simulink library "tqd"  (R2021b)
settings: Solver=VariableStepAuto  StartTime=0.0  StopTime=10.0  RelTol=1e-3
undefined symbols (not defined in the file or in its folder): ATQD_AccelLimitInRange_X_rpm, ATQD_AccelLimitInRange_Y_Nm, ATQD_AccelLimitOvrKi_X_Nm, ATQD_AccelLimitOvrKp_X_Nm, ATQD_BOSMapD_X_rpm, ATQD_BOSMapD_Y_pct, ATQD_BOSMapR_X_rpm, ATQD_BOSMapR_Y_pct, ATQD_HVBCurrSmooth_X_A, ATQD_LHMTqMapDLC_X_rpm, ATQD_LHMTqMapDLC_Y_pct, ATQD_LHMTqMapRLC_X_rpm, ATQD_LHMTqMapRLC_Y_pct, ATQD_NormalMapDLC_X_rpm, ATQD_NormalMapDLC_Y_pct, ATQD_NormalTqDecSR_X_rpm, ATQD_NormalTqDecSR_Y_Nm, ATQD_NormalTqIncSR_X_rpm, ATQD_NormalTqIncSR_Y_Nm, ATQD_OPDMapRLC_X_rpm, ATQD_OPDMapRLC_Y_pct, ATQD_RollRegTorReq_X_rpm, ATQD_RollRegTorReq_Y_enum, ATQD_VehSpdLimitInRange_X_rpm, ATQD_VehSpdLimitInRange_Y_Nm, ATQD_VehSpdLimitOvrKi_X_Nm, ATQD_VehSpdLimitOvrKp_X_Nm, EIGHT_INT, ENUM_BRAKEPEDAL_PRESSED, ENUM_BRAKEPEDAL_RELEASED, ENUM_COMBOKEY_DOWN, ENUM_COMBOKEY_M1, ENUM_COMBOKEY_M2, ENUM_COMBOKEY_NONE, ENUM_COMBOKEY_RKNEE, ENUM_COMBOKEY_STOPLV, ENUM_COMBOKEY_UP, ENUM_CP2VKNEEREQ_REQUEST, ENUM_CP2VNLVREQ_LEVEL1, ENUM_CP2VNLVREQ_LEVEL2, ENUM_CP2VNLVREQ_LOWER, ENUM_CP2VNLVREQ_STOPLV, ENUM_CP2VNLVREQ_UPPER, ENUM_CREEPIND_DISABLE, ENUM_CREEPIND_READY, ENUM_CREEPIND_RUNNING, ENUM_CREEPIND_WARNING, ENUM_DRIVELINERELEASE_RELEASE, ENUM_EBSTORQUERWQ_LIMIT, ENUM_EBSTORQUERWQ_TORQUE, ENUM_ECPVCUDRM_CONFORT, ENUM_ECPVCUDRM_ECO, ENUM_ECPVCUDRM_NORMAL, ENUM_ECPVCUDRM_NOTAVAILABLE, ENUM_EMTqModeDrvBrk_Accel, ENUM_EMTqModeDrvBrk_Brake, ENUM_EMTqModeDrvBrk_Coast, ENUM_ETC2ACTDRIVEDIR_BACKWARD, ENUM_ETC2ACTDRIVEDIR_FORWARD, ENUM_ETC2ACTDRIVEDIR_STILL ... (+341)
libraries: simulink x109, hcu_lib x67
(part 1 of 13)
settings Model: Creator=13615  LastModifiedBy=zack
settings SolverCC: AlgebraicLoopSolver=TrustRegion
settings DataIOCC: SaveFormat=Array  SignalLoggingSaveFormat=ModelDataLogs  ReturnWorkspaceOutputs=off
settings OptimizationCC: BlockReduction=off  BooleanDataType=off
settings DebuggingCC: SaveWithParameterizedLinksMsg=none  UnderspecifiedInitializationDetection=Classic  MergeDetectMultiDrivingBlocksExec=none  SignalResolutionControl=TryResolveAllWithWarning
settings HardwareCC: TargetUnknown=on
settings ModelReferenceCC: PropagateSignalLabelsOutOfModel=off
settings SFSimCC: SimUseLocalCustomCode=off
settings RTWCC: RTWUseLocalCustomCode=off
settings ConfigComp: CovMetricSettings=dw  CovSaveCumulativeToWorkspaceVar=on  CovSaveSingleToWorkspaceVar=on

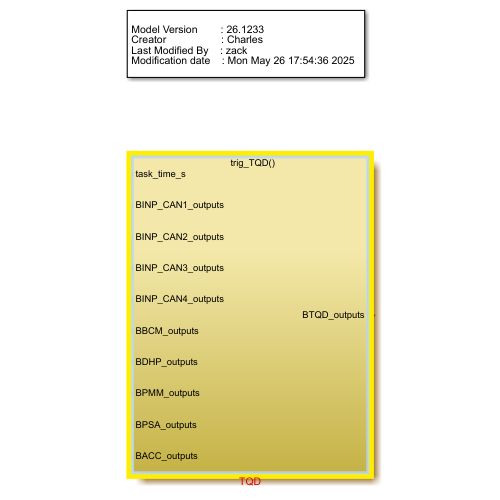
[thumbnail: Simulink's stored preview of the top-level diagram]
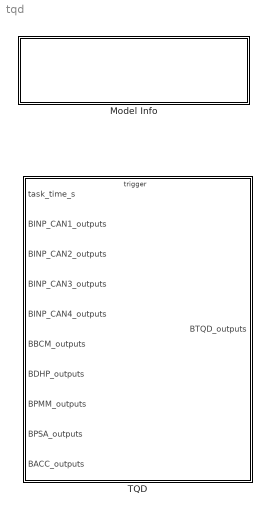
== system tqd ==
  Model Info : Subsystem  LoadFcn=slcm LoadBlock;  InitFcn=slcm('UpdateAllCMBlocksInThisModelInit')  mask(CMBlock){InitialSaveTempField=, InitialBlockCM=None, BlockCM=None, Frame=on, SaveTempField=, DisplayStringWithTags=|, MaskDisplayString=Model Version        : 26.1236\nCreator                   : Charles\nLast Modified By    : zack\nModification date    : Mon May 26 18:16:00 2025, HorizontalTextAlignment=Left, LeftAlignmentValue=0.02, SourceBlockDiagram=tqd, TagMaxNumber=20, CMTag1=, CMTag2=, CMTag3=, CMTag4=, CMTag5=, CMTag6=, CMTag7=, CMTag8=, CMTag9=, CMTag10=, CMTag11=, CMTag12=, CMTag13=, CMTag14=, CMTag15=, CMTag16=, CMTag17=, CMTag18=, CMTag19=, CMTag20=}
      mask DisplayStringWithTags=|
      | Model Version        : %<ModelVersion>
      | Creator                   : Charles
      | Last Modified By    : %<LastModifiedBy>
      | Modification date    : %<LastModificationDate>
      mask help: This block allows revision control information to be displayed within the model.
      settings: CopyFcn=slcm CopyBlock;  DeleteFcn=slcm Cancel;  PostSaveFcn=slcm('UpdateAllCMBlocksInThisModel')  NameChangeFcn=slcm Rename;  OpenFcn=slcm
      mask Display: text(str2num(LeftAlignmentValue), 0.5, MaskDisplayString, 'HorizontalAlignment', HorizontalTextAlignment)
  TQD : Subsystem
      settings: RTWSystemCode=Nonreusable function  RTWFcnNameOpts=Use subsystem name  RTWFileNameOpts=Use subsystem name

== system tqd/Model Info ==
  EmptySubsystem : Subsystem

== system tqd/TQD ==
  task_time_s : Inport  OutDataTypeStr=single
  BINP_CAN1_outputs : Inport  Port=2  OutDataTypeStr=Bus:BINP_CAN1_outputs
  BINP_CAN2_outputs : Inport  Port=3  OutDataTypeStr=Bus: BINP_CAN2_outputs
  BINP_CAN3_outputs : Inport  Port=4  OutDataTypeStr=Bus:BINP_CAN3_outputs
  BINP_CAN4_outputs : Inport  Port=5  OutDataTypeStr=Bus:BINP_CAN4_outputs
  BBCM_outputs : Inport  Port=6  OutDataTypeStr=Bus:BBCM_outputs
  BDHP_outputs : Inport  Port=7  OutDataTypeStr=Bus:BDHP_outputs
  BPMM_outputs : Inport  Port=8  OutDataTypeStr=Bus:BPMM_outputs
  BPSA_outputs : Inport  Port=9  OutDataTypeStr=Bus:BPSA_outputs
  BACC_outputs : Inport  Port=10  OutDataTypeStr=Bus:BACC_outputs
  trig_TQD : TriggerPort  TriggerType=function-call  VariantControl=(inherit)
  Input_Convert : Subsystem
      settings: RTWSystemCode=Nonreusable function
  Main : Subsystem
      settings: RTWSystemCode=Nonreusable function
  OutpConvert : Subsystem
      settings: RTWSystemCode=Nonreusable function
  SCP_In : Subsystem
      settings: RTWSystemCode=Nonreusable function
  SCP_Out : Subsystem
      settings: RTWSystemCode=Nonreusable function
  BTQD_outputs : Outport  OutDataTypeStr=Bus:BTQD_outputs
  wires:
  task_time_s/1 -> SCP_In/1(task_time_s)
  BINP_CAN1_outputs/1 -> SCP_In/2(BINP_CAN1_outputs)
  BINP_CAN2_outputs/1 -> SCP_In/3(BINP_CAN2_outputs)
  BINP_CAN3_outputs/1 -> SCP_In/4(BINP_CAN3_outputs)
  BINP_CAN4_outputs/1 -> SCP_In/5(BINP_CAN4_outputs)
  BBCM_outputs/1 -> SCP_In/6(BBCM_outputs)
  BDHP_outputs/1 -> SCP_In/7(BDHP_outputs)
  BPMM_outputs/1 -> SCP_In/8(BPMM_outputs)
  BPSA_outputs/1 -> SCP_In/9(BPSA_outputs)
  SCP_In/1(BSCPIn_outputs) -> [BSCPIn_outputs]
  [BSCPIn_outputs] -> Input_Convert/1(BSCPIn_outputs)
  [BMain_outputs] -> Input_Convert/2(BMain_outputs)
  Input_Convert/1(BInpConvert_outputs) -> [BInpConvert_outputs]
  [BInpConvert_outputs] -> Main/2(BInpConvert_outputs)
  [BSCPIn_outputs] -> Main/1(BSCPIn_outputs)
  Main/1(BMain_outputs) -> [BMain_outputs]
  [BSCPIn_outputs] -> OutpConvert/1(BSCPIn_outputs)
  [BInpConvert_outputs] -> OutpConvert/2(BInpConvert_outputs)
  [BMain_outputs] -> OutpConvert/3(BMain_outputs)
  OutpConvert/1(BOutpConvert_outputs) -> [BOutpConvert_outputs]
  [BMain_outputs] -> SCP_Out/2(BMain_outputs)
  [BOutpConvert_outputs] -> SCP_Out/3(BOutpConvert_outputs)
  [BInpConvert_outputs] -> SCP_Out/1(BInpConvert_outputs)
  SCP_Out/1(BTQD_outputs) -> BTQD_outputs/1
  BACC_outputs/1 -> SCP_In/10(BACC_outputs)

== system tqd/Model Info/EmptySubsystem ==

== system tqd/TQD/Input_Convert ==
  BSCPIn_outputs : Inport
  BMain_outputs : Inport  Port=2
  Bus Creator : BusCreator  Inputs=101
  Bus Selector : BusSelector  OutputSignals=VTQD_AccelPedalDepressed_flg,VTQD_BrkSWOn_flg,VTQD_DoorOpen_flg,VTQD_DrivePositionOn_flg,VTQD_NeutralPositionOn_flg,VTQD_ReversePositionOn_flg,VTQD_EVDriveReady_flg,VTQD_IGNActive_flg,VTQD_EM1ReqTorqLimDriv_Nm,VTQD_EM1ReqTorqLimBrk_Nm,VTQD_ActFRDoorOPSta_flg,VTQD_ActMDDoorOPSta_flg,VTQD_ActTDDoorOPSta_flg,VTQD_VCU4PweLmtInd_flg,VTQD_GearFlashIndDis_flg,VTQD_GearFlashInd_flg,VTQD_EVCU1VehActDrvDir_enum,VTQD_VCUMCUDemHiPosVal_rpm,VTQD_SpdLimSta_flg,VTQD_EngModeEnDetTime_s,VTQD_EngModeEnDetEnd_flg,VTQD_LVchrgSvrMode_flg,VTQD_EngModeDisDetTime_s,VTQD_EngModeDisDetEnd_flg,VTQD_AmberFlashOn_flg,VTQD_AmberFlashOff_flg,VTQD_Function1Off_flg,VTQD_Function2Off_flg,VTQD_Function3Off_flg,VTQD_Function4Off_flg,VTQD_Function5Off_flg,VTQD_ComboKeyEn_flg,VTQD_ComboKeyPreEn_flg,VTQD_FunctionOffSta_enum,VTQD_LostComBCU_flg,VTQD_LostComDMS_flg,VTQD_LostComEBS_flg,VTQD_LostComTempEBS_flg,VTQD_LostComTempMCU_flg,VTQD_LostComTempBCU_flg,VTQD_SpdForceZero_flg,VTQD_TrqForceZero_flg,VTQD_TrqLimit_flg,VTQD_SpdLimit_flg,VTQD_DMSLossLimitGear_flg,VTQD_DRTransfer_flg,VTQD_TMRotateDirectionReq_enum,VTQD_ActvDmpDisabReq_flg,VTQD_ForceDischarge_flg,VTQD_TqTargetShaftSpd_rpm,VTQD_PTAvailMotTq_Nm,VTQD_PTAvailGenTq_Nm,VTQD_ActDriveMode_enum,VTQD_ComLostZeroPwr_flg,VTQD_EBSLostZeroReg_flg,VTQD_ActCAN1BUSOFF_flg,VTQD_EM1LimitCtrlBrk_flg,VTQD_EM1TorqueCtrlBrk_flg,VTQD_EM1TorqueCtrlDriv_flg,VTQD_EM1LimitCtrlDriv_flg,VTQD_TrqCMDForveZero_flg,VTQD_TqSource_enum,VTQD_TMSpd_rpm,VTQD_VCUTMVehSpd_kph,VTQD_VCUVehSpd_kph
  Bus Selector1 : BusSelector  OutputSignals=VTQD_GearActualPosn_enum,VTQD_ParkingPawlPwrOn_flg,VTQD_ParkingPawlEnable_flg,VTQD_TorqLimDoorOpn_flg,VTQD_VCUMCUCtrlMdTQD_enum,VTQD_PedalMapTq_Nm,VTQD_BOSTqDecRate_pct,VTQD_CreepSpdReq_rpm,VTQD_CreepStart_flg,VTQD_CreepIND_enum,VTQD_ActTUpAIND_enum,VTQD_VCUEBSHHSw_enum,VTQD_VCUEBSRd4BR_enum,VTQD_TUpADisableCreep_flg,VTQD_RollingRegenEnable_flg,VTQD_RollRegTorReq_Nm,VTQD_VehSpdLimitEnable_flg,VTQD_VehSpdLimitTG_kph,VTQD_VehSpdTorLimit_Nm,VTQD_VehAcclLimitEnable_flg,VTQD_VehAcclLimitTG_mps2,VTQD_VehAcclTorLimit_Nm,VTQD_VehAccel_mps2,VTQD_ParkingProtectWarning_flg,VTQD_ParkingProtectAction_flg,VTQD_TqCMDUpLim_Nm,VTQD_TqCMDLowLim_Nm,VTQD_RampTs_c,VTQD_RampTqIncSR_Nm,VTQD_RampTqDecSR_Nm,VTQD_FrEDUSpRat_rat,VTQD_RrEDUSpRat_rat,VTQD_FinalTrqUpLim_Nm,VTQD_FinalTrqLowLim_Nm,VTQD_TMTqCapMot_Nm,VTQD_TMTqCapGen_Nm
  Function : Subsystem
      settings: RTWSystemCode=Nonreusable function
  Input Signal Convert : Subsystem
      settings: RTWSystemCode=Nonreusable function
  BInpConvert_outputs : Outport
  wires:
  BSCPIn_outputs/1 -> [BSCPIn_outputs]
  BMain_outputs/1 -> [BMain_outputs]
  [BSCPIn_outputs] -> Input Signal Convert/1(BSCPIn_outputs)
  Input Signal Convert/1(BSignalConvert_outputs) -> [BSignalConvert_outputs]
  [BSCPIn_outputs] -> Function/1(BSCPIn_outputs)
  [BSignalConvert_outputs] -> Function/2(BSignalConvert_outputs)
  [BMain_outputs] -> Input Signal Convert/3(BDCQ_main_outputs)
  [BMain_outputs] -> Function/3(BMain_outputs)
  Function/1(BFunction_outputs) -> [BFunction_outputs]
  [BFunction_outputs] -> Input Signal Convert/2(BDCQ_Function_outputs)
  [BSignalConvert_outputs] -> Bus Selector/1
  [BFunction_outputs] -> Bus Selector1/1
  Bus Selector/1 -> Bus Creator/1  "<VTQD_AccelPedalDepressed_flg>"
  Bus Selector/2 -> Bus Creator/2  "<VTQD_BrkSWOn_flg>"
  Bus Selector/3 -> Bus Creator/3  "<VTQD_DoorOpen_flg>"
  Bus Selector/4 -> Bus Creator/4  "<VTQD_DrivePositionOn_flg>"
  Bus Selector/5 -> Bus Creator/5  "<VTQD_NeutralPositionOn_flg>"
  Bus Selector/6 -> Bus Creator/6  "<VTQD_ReversePositionOn_flg>"
  Bus Selector/7 -> Bus Creator/7  "<VTQD_EVDriveReady_flg>"
  Bus Selector/8 -> Bus Creator/8  "<VTQD_IGNActive_flg>"
  Bus Selector/9 -> Bus Creator/9  "<VTQD_EM1ReqTorqLimDriv_Nm>"
  Bus Selector/10 -> Bus Creator/10  "<VTQD_EM1ReqTorqLimBrk_Nm>"
  Bus Selector/11 -> Bus Creator/11  "<VTQD_ActFRDoorOPSta_flg>"
  Bus Selector/12 -> Bus Creator/12  "<VTQD_ActMDDoorOPSta_flg>"
  Bus Selector/13 -> Bus Creator/13  "<VTQD_ActTDDoorOPSta_flg>"
  Bus Selector/14 -> Bus Creator/14  "<VTQD_VCU4PweLmtInd_flg>"
  Bus Selector/15 -> Bus Creator/15  "<VTQD_GearFlashIndDis_flg>"
  Bus Selector/16 -> Bus Creator/16  "<VTQD_GearFlashInd_flg>"
  Bus Selector/17 -> Bus Creator/17  "<VTQD_EVCU1VehActDrvDir_enum>"
  Bus Selector/18 -> Bus Creator/18  "<VTQD_VCUMCUDemHiPosVal_rpm>"
  Bus Selector/19 -> Bus Creator/19  "<VTQD_SpdLimSta_flg>"
  Bus Selector/20 -> Bus Creator/20  "<VTQD_EngModeEnDetTime_s>"
  Bus Selector/21 -> Bus Creator/21  "<VTQD_EngModeEnDetEnd_flg>"
  Bus Selector/22 -> Bus Creator/22  "<VTQD_LVchrgSvrMode_flg>"
  Bus Selector/23 -> Bus Creator/23  "<VTQD_EngModeDisDetTime_s>"
  Bus Selector/24 -> Bus Creator/24  "<VTQD_EngModeDisDetEnd_flg>"
  Bus Selector/25 -> Bus Creator/25  "<VTQD_AmberFlashOn_flg>"
  Bus Selector/26 -> Bus Creator/26  "<VTQD_AmberFlashOff_flg>"
  Bus Selector/27 -> Bus Creator/27  "<VTQD_Function1Off_flg>"
  Bus Selector/28 -> Bus Creator/28  "<VTQD_Function2Off_flg>"
  Bus Selector/29 -> Bus Creator/29  "<VTQD_Function3Off_flg>"
  Bus Selector/30 -> Bus Creator/30  "<VTQD_Function4Off_flg>"
  Bus Selector/31 -> Bus Creator/31  "<VTQD_Function5Off_flg>"
  Bus Selector/32 -> Bus Creator/32  "<VTQD_ComboKeyEn_flg>"
  Bus Selector/33 -> Bus Creator/33  "<VTQD_ComboKeyPreEn_flg>"
  Bus Selector/34 -> Bus Creator/34  "<VTQD_FunctionOffSta_enum>"
  Bus Selector/35 -> Bus Creator/35  "<VTQD_LostComBCU_flg>"
  Bus Selector/36 -> Bus Creator/36  "<VTQD_LostComDMS_flg>"
  Bus Selector/37 -> Bus Creator/37  "<VTQD_LostComEBS_flg>"
  Bus Selector/38 -> Bus Creator/38  "<VTQD_LostComTempEBS_flg>"
  Bus Selector/39 -> Bus Creator/39  "<VTQD_LostComTempMCU_flg>"
  Bus Selector/40 -> Bus Creator/40  "<VTQD_LostComTempBCU_flg>"
  Bus Selector/41 -> Bus Creator/41  "<VTQD_SpdForceZero_flg>"
  Bus Selector/42 -> Bus Creator/42  "<VTQD_TrqForceZero_flg>"
  Bus Selector/43 -> Bus Creator/43  "<VTQD_TrqLimit_flg>"
  Bus Selector/44 -> Bus Creator/44  "<VTQD_SpdLimit_flg>"
  Bus Selector/45 -> Bus Creator/45  "<VTQD_DMSLossLimitGear_flg>"
  Bus Selector/46 -> Bus Creator/46  "<VTQD_DRTransfer_flg>"
  Bus Selector/47 -> Bus Creator/47  "<VTQD_TMRotateDirectionReq_enum>"
  Bus Selector/48 -> Bus Creator/48  "<VTQD_ActvDmpDisabReq_flg>"
  Bus Selector/49 -> Bus Creator/49  "<VTQD_ForceDischarge_flg>"
  Bus Selector/50 -> Bus Creator/50  "<VTQD_TqTargetShaftSpd_rpm>"
  Bus Selector/51 -> Bus Creator/51  "<VTQD_PTAvailMotTq_Nm>"
  Bus Selector/52 -> Bus Creator/52  "<VTQD_PTAvailGenTq_Nm>"
  Bus Selector/53 -> Bus Creator/53  "<VTQD_ActDriveMode_enum>"
  Bus Selector/54 -> Bus Creator/54  "<VTQD_ComLostZeroPwr_flg>"
  Bus Selector/55 -> Bus Creator/55  "<VTQD_EBSLostZeroReg_flg>"
  Bus Selector/56 -> Bus Creator/56  "<VTQD_ActCAN1BUSOFF_flg>"
  Bus Selector/57 -> Bus Creator/57  "<VTQD_EM1LimitCtrlBrk_flg>"
  Bus Selector/58 -> Bus Creator/58  "<VTQD_EM1TorqueCtrlBrk_flg>"
  Bus Selector/59 -> Bus Creator/59  "<VTQD_EM1TorqueCtrlDriv_flg>"
  Bus Selector/60 -> Bus Creator/60  "<VTQD_EM1LimitCtrlDriv_flg>"
  Bus Selector/61 -> Bus Creator/61  "<VTQD_TrqCMDForveZero_flg>"
  Bus Selector/62 -> Bus Creator/62  "<VTQD_TqSource_enum>"
  Bus Selector/63 -> Bus Creator/63  "<VTQD_TMSpd_rpm>"
  Bus Selector/64 -> Bus Creator/64  "<VTQD_VCUTMVehSpd_kph>"
  Bus Selector/65 -> Bus Creator/65  "<VTQD_VCUVehSpd_kph>"
  Bus Selector1/9 -> Bus Creator/74  "<VTQD_CreepStart_flg>"
  Bus Selector1/8 -> Bus Creator/73  "<VTQD_CreepSpdReq_rpm>"
  Bus Selector1/10 -> Bus Creator/75  "<VTQD_CreepIND_enum>"
  Bus Selector1/7 -> Bus Creator/72  "<VTQD_BOSTqDecRate_pct>"
  Bus Selector1/11 -> Bus Creator/76  "<VTQD_ActTUpAIND_enum>"
  Bus Selector1/6 -> Bus Creator/71  "<VTQD_PedalMapTq_Nm>"
  Bus Selector1/12 -> Bus Creator/77  "<VTQD_VCUEBSHHSw_enum>"
  Bus Selector1/5 -> Bus Creator/70  "<VTQD_VCUMCUCtrlMdTQD_enum>"
  Bus Selector1/13 -> Bus Creator/78  "<VTQD_VCUEBSRd4BR_enum>"
  Bus Selector1/4 -> Bus Creator/69  "<VTQD_TorqLimDoorOpn_flg>"
  Bus Selector1/14 -> Bus Creator/79  "<VTQD_TUpADisableCreep_flg>"
  Bus Selector1/3 -> Bus Creator/68  "<VTQD_ParkingPawlEnable_flg>"
  Bus Selector1/15 -> Bus Creator/80  "<VTQD_RollingRegenEnable_flg>"
  Bus Selector1/2 -> Bus Creator/67  "<VTQD_ParkingPawlPwrOn_flg>"
  Bus Selector1/16 -> Bus Creator/81  "<VTQD_RollRegTorReq_Nm>"
  Bus Selector1/1 -> Bus Creator/66  "<VTQD_GearActualPosn_enum>"
  Bus Selector1/17 -> Bus Creator/82  "<VTQD_VehSpdLimitEnable_flg>"
  Bus Selector1/18 -> Bus Creator/83  "<VTQD_VehSpdLimitTG_kph>"
  Bus Selector1/19 -> Bus Creator/84  "<VTQD_VehSpdTorLimit_Nm>"
  Bus Selector1/20 -> Bus Creator/85  "<VTQD_VehAcclLimitEnable_flg>"
  Bus Selector1/21 -> Bus Creator/86  "<VTQD_VehAcclLimitTG_mps2>"
  Bus Selector1/22 -> Bus Creator/87  "<VTQD_VehAcclTorLimit_Nm>"
  Bus Selector1/23 -> Bus Creator/88  "<VTQD_VehAccel_mps2>"
  Bus Selector1/24 -> Bus Creator/89  "<VTQD_ParkingProtectWarning_flg>"
  Bus Selector1/25 -> Bus Creator/90  "<VTQD_ParkingProtectAction_flg>"
  Bus Selector1/26 -> Bus Creator/91  "<VTQD_TqCMDUpLim_Nm>"
  Bus Selector1/27 -> Bus Creator/92  "<VTQD_TqCMDLowLim_Nm>"
  Bus Selector1/28 -> Bus Creator/93  "<VTQD_RampTs_c>"
  Bus Selector1/29 -> Bus Creator/94  "<VTQD_RampTqIncSR_Nm>"
  Bus Selector1/30 -> Bus Creator/95  "<VTQD_RampTqDecSR_Nm>"
  Bus Selector1/31 -> Bus Creator/96  "<VTQD_FrEDUSpRat_rat>"
  Bus Selector1/32 -> Bus Creator/97  "<VTQD_RrEDUSpRat_rat>"
  Bus Selector1/33 -> Bus Creator/98  "<VTQD_FinalTrqUpLim_Nm>"
  Bus Selector1/34 -> Bus Creator/99  "<VTQD_FinalTrqLowLim_Nm>"
  Bus Selector1/35 -> Bus Creator/100  "<VTQD_TMTqCapMot_Nm>"
  Bus Selector1/36 -> Bus Creator/101  "<VTQD_TMTqCapGen_Nm>"
  Bus Creator/1 -> BInpConvert_outputs/1  "BInpConvert_outputs"

== system tqd/TQD/Main ==
  BSCPIn_outputs : Inport
  BInpConvert_outputs : Inport  Port=2
  Available Torqeu Limitation : Subsystem
      settings: RTWSystemCode=Nonreusable function
  Bus Creator : BusCreator  Inputs=9
  Driver Torque Demmand : Subsystem
      settings: RTWSystemCode=Nonreusable function
  Gear Ratio : Subsystem
  Motor Direction : Subsystem
      settings: RTWSystemCode=Nonreusable function
  Ramp Input Torque : Subsystem
      settings: RTWSystemCode=Nonreusable function
  Torque Coordination : Subsystem
      settings: RTWSystemCode=Nonreusable function
  Torque Distribution : Subsystem
      settings: RTWSystemCode=Nonreusable function
  Torque Ramp : Subsystem
      settings: RTWSystemCode=Nonreusable function
  BMain_outputs : Outport
  wires:
  [VTQD_TMTqReq_Nm] -> Bus Creator/9
  Ramp Input Torque/1(VTQD_RrRampInpTqRr_Nm) -> [VTQD_RrRampInpTqRr_Nm]
  [VTQD_RrRampInpTqRr_Nm] -> Torque Ramp/3(VTQD_RrRampInpTqRr_Nm)
  [BInpConvert_outputs] -> Torque Distribution/1(BInpConvert_outputs)
  Torque Distribution/1(VTQD_CoorTqDemFr_Nm) -> [VTQD_CoorTqDemFr_Nm]
  [BSCPIn_outputs] -> Available Torqeu Limitation/2(BSCPIn_outputs)
  Bus Creator/1 -> BMain_outputs/1  "BMain_outputs"
  [VTQD_AfterAvailableTqDemRr_Nm] -> Bus Creator/5
  [VTQD_DriverTqDem_Nm] -> Torque Coordination/2(VTQD_DriverTqDem_Nm)
  [VTQD_TMTqReqRaw_Nm] -> Motor Direction/2(VTQD_TMTqReqRaw_Nm)
  [BInpConvert_outputs] -> Ramp Input Torque/1(BInpConvert_outputs)
  Motor Direction/1(VTQD_TMTqReq_Nm) -> [VTQD_TMTqReq_Nm]
  Torque Ramp/2(VTQD_RrRampTq_Nm) -> [VTQD_RrRampTq_Nm]
  [BSCPIn_outputs] -> Ramp Input Torque/2(BSCPIn_outputs)
  Torque Distribution/2(VTQD_CoorTqDemRr_Nm) -> [VTQD_CoorTqDemRr_Nm]
  Torque Ramp/1(VTQD_TMTqReqRaw_Nm) -> [VTQD_TMTqReqRaw_Nm]
  [VTQD_CoordTqDem_Nm] -> Bus Creator/2
  [BInpConvert_outputs] -> Motor Direction/1(BInpConvert_outputs)
  [VTQD_RrRampInpTqRr_Nm] -> Bus Creator/6
  [VTQD_RrRampTq_Nm] -> Bus Creator/8
  [VTQD_DriverTqDem_Nm] -> Bus Creator/1
  [VTQD_CoorTqDemRr_Nm] -> Available Torqeu Limitation/3(VTQD_CoorTqDemRr_Nm)
  [VTQD_CoorTqDemRr_Nm] -> Bus Creator/4
  BSCPIn_outputs/1 -> [BSCPIn_outputs]
  [BInpConvert_outputs] -> Torque Coordination/1(BInpConvert_outputs)
  Torque Coordination/1(VTQD_CoordTqDem_Nm) -> [VTQD_CoordTqDem_Nm]
  [BInpConvert_outputs] -> Driver Torque Demmand/1(BDCQ_InpConvert_outputs)
  [BInpConvert_outputs] -> Available Torqeu Limitation/1(BInpConvert_outputs)
  Driver Torque Demmand/1(VTQD_DriverTqDem_Nm) -> [VTQD_DriverTqDem_Nm]
  BInpConvert_outputs/1 -> [BInpConvert_outputs]
  [VTQD_CoordTqDem_Nm] -> Torque Distribution/2(VTQD_CoordTqDem_Nm)
  [VTQD_AfterAvailableTqDemRr_Nm] -> Ramp Input Torque/3(VTQD_AfterAvailableTqDemRr_Nm)
  [BInpConvert_outputs] -> Torque Ramp/1(BInpConvert_outputs)
  Available Torqeu Limitation/1(VTQD_AfterAvailableTqDemRr_Nm) -> [VTQD_AfterAvailableTqDemRr_Nm]
  [VTQD_CoorTqDemFr_Nm] -> Bus Creator/3
  [VTQD_TMTqReqRaw_Nm] -> Bus Creator/7
  [BSCPIn_outputs] -> Torque Ramp/2(BSCPIn_outputs)

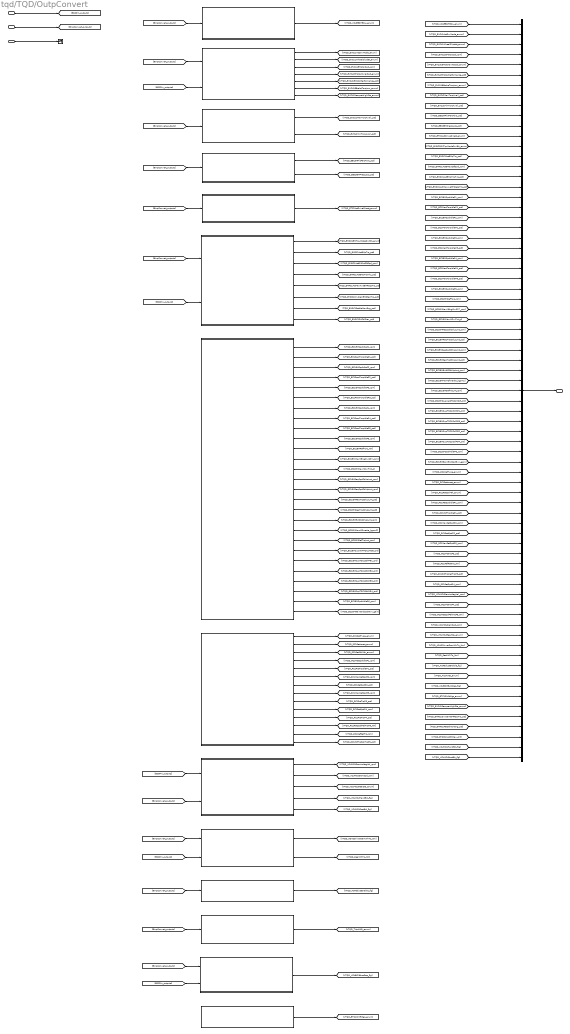
== system tqd/TQD/OutpConvert ==
  BSCPIn_outputs : Inport
  BInpConvert_outputs : Inport  Port=2
  BMain_outputs : Inport  Port=3
  ABS_System_Enable : Subsystem
      settings: RTWSystemCode=Nonreusable function
  ADAS_DriverWheelTqDem : Subsystem
      settings: RTWSystemCode=Nonreusable function
  Bus Creator : BusCreator  Inputs=73
  Buzzer Request : Subsystem
      settings: RTWSystemCode=Nonreusable function
  EC1 SCP : Subsystem
      settings: RTWSystemCode=Nonreusable function
  EEC3 SCP : Subsystem
      settings: RTWSystemCode=Nonreusable function
  EMRC1 SCP : Subsystem
      settings: RTWSystemCode=Nonreusable function
  ETC1 SCP : Subsystem
      settings: RTWSystemCode=Nonreusable function
  ETC2 SCP : Subsystem
      settings: RTWSystemCode=Nonreusable function
  EVCU1 SCP : Subsystem
      settings: RTWSystemCode=Nonreusable function
  EVCU2 SCP : Subsystem
      settings: RTWSystemCode=Nonreusable function
  MCUCMD SCP : Subsystem
      settings: RTWSystemCode=Nonreusable function
  MSF SCP : Subsystem
      settings: RTWSystemCode=Nonreusable function
  RC1 SCP : Subsystem
      settings: RTWSystemCode=Nonreusable function
  TUpA Indication : Subsystem
      settings: RTWSystemCode=Nonreusable function
  Terminator : Terminator
  BOutpConvert_outputs : Outport
  wires:
  [VTQD_EC1PercTorqIdleP4_pct] -> Bus Creator/25
  [BSCPIn_outputs] -> EVCU1 SCP/2(BSCPIn_outputs)
  [VTQD_RC1RetSpdP4_rpm] -> Bus Creator/56
  [VTQD_EC1EMGainEndSpdGvn_gain] -> Bus Creator/44
  MSF SCP/1(VTQD_VCUEBSHBSw_enum) -> [VTQD_VCUEBSHBSw_enum]
  [VTQD_EVCU2MaxTorqAvail_pct] -> Bus Creator/8
  EVCU1 SCP/4(VTQD_EVCU1EMotorOvrerSpd_enum) -> [VTQD_EVCU1EMotorOvrerSpd_enum]
  BInpConvert_outputs/1 -> [BInpConvert_outputs]
  EVCU1 SCP/2(VTQD_EVCU1WheelSlipdet_enum) -> [VTQD_EVCU1WheelSlipdet_enum]
  [VTQD_EC1EMSpdIdleP5_rpm] -> Bus Creator/27
  [BInpConvert_outputs] -> MSF SCP/1(BInpConvert_outputs)
  [BInpConvert_outputs] -> ETC2 SCP/1(BInpConvert_outputs)
  [VTQD_EC1EMSupTSC1CtrlPG2_cnt] -> Bus Creator/41
  [BInpConvert_outputs] -> EVCU1 SCP/1(BInpConvert_outputs)
  EC1 SCP/13(VTQD_EC1EMMaxMOvrTmt_s) -> [VTQD_EC1EMMaxMOvrTmt_s]
  [VTQD_RealWhTq_Nm] -> Bus Creator/63
  EVCU1 SCP/1(VTQD_EVCU1ActDrvMode_enum) -> [VTQD_EVCU1ActDrvMode_enum]
  [VTQD_EC1EMSupTSC1CtrlPG3_cnt] -> Bus Creator/40
  BSCPIn_outputs/1 -> [BSCPIn_outputs]
  [BInpConvert_outputs] -> EVCU2 SCP/1(BInpConvert_outputs)
  [VTQD_EVCU1WheelSlipdet_enum] -> Bus Creator/3
  EVCU1 SCP/3(VTQD_EVCU1EMotorSpd_rpm) -> [VTQD_EVCU1EMotorSpd_rpm]
  [BSCPIn_outputs] -> EMRC1 SCP/2(BSCPIn_outputs)
  [VTQD_VCUMCUDemLoNegVal_rpm] -> Bus Creator/57
  EC1 SCP/10(VTQD_EC1EMSpdIdleP5_rpm) -> [VTQD_EC1EMSpdIdleP5_rpm]
  [BInpConvert_outputs] -> EEC3 SCP/1(BInpConvert_outputs)
  [VTQD_EC1EMReqSpdCtrlUpLmt_rpm] -> Bus Creator/33
  [VTQD_EC1EMSpdIdleP2_rpm] -> Bus Creator/20
  EC1 SCP/25(VTQD_EC1EMSupTSC1CtrlPG4_cnt) -> [VTQD_EC1EMSupTSC1CtrlPG4_cnt]
  EMRC1 SCP/3(VTQD_EMRC1ActEMOutSftSpd_rpm) -> [VTQD_EMRC1ActEMOutSftSpd_rpm]
  RC1 SCP/14(VTQD_RC1PctTrqPekTrqP5_pct) -> [VTQD_RC1PctTrqPekTrqP5_pct]
  EC1 SCP/7(VTQD_EC1EMSpdIdleP4_rpm) -> [VTQD_EC1EMSpdIdleP4_rpm]
  EEC3 SCP/1(VTQD_EEC3NFricPercTorq_pct) -> [VTQD_EEC3NFricPercTorq_pct]
  EC1 SCP/22(VTQD_EC1EMSupTSC1CtrlPG1_cnt) -> [VTQD_EC1EMSupTSC1CtrlPG1_cnt]
  EEC3 SCP/2(VTQD_EEC3EMPressLoss_pct) -> [VTQD_EEC3EMPressLoss_pct]
  EMRC1 SCP/1(VTQD_EMRC1EMTquModeDrvBrk_enum) -> [VTQD_EMRC1EMTquModeDrvBrk_enum]
  [VTQD_EC1EMMaxMOvrTmt_s] -> Bus Creator/30
  [VTQD_EC1EMExtRSCtrlUpLmt_rpm] -> Bus Creator/35
  EC1 SCP/1(VTQD_EC1EMSpdIdleP1_rpm) -> [VTQD_EC1EMSpdIdleP1_rpm]
  [VTQD_EVCU1EMotorOvrerSpd_enum] -> Bus Creator/5
  [BInpConvert_outputs] -> EMRC1 SCP/1(BInpConvert_outputs)
  [BSCPIn_outputs] -> MCUCMD SCP/1(BSCPIn_outputs)
  EMRC1 SCP/2(VTQD_EMRC1ActEMpTrq_pct) -> [VTQD_EMRC1ActEMpTrq_pct]
  EVCU1 SCP/5(VTQD_EVCU1EMotorPerformance_pct) -> [VTQD_EVCU1EMotorPerformance_pct]
  [VTQD_RC1MaxRetSpdP3_rpm] -> Bus Creator/52
  [VTQD_RC1RetLocat_enum] -> Bus Creator/46
  [VTQD_ETC2ActDriveDirect_enum] -> Bus Creator/12
  EC1 SCP/3(VTQD_EC1EMSpdIdleP2_rpm) -> [VTQD_EC1EMSpdIdleP2_rpm]
  [VTQD_EC1PercTorqIdleP2_pct] -> Bus Creator/21
  [VTQD_RC1RetSpdP2_pct] -> Bus Creator/51
  [VTQD_EC1EMSpdIdleP3_rpm] -> Bus Creator/22
  EC1 SCP/14(VTQD_EC1EMReqSpdCtrlLoLmt_rpm) -> [VTQD_EC1EMReqSpdCtrlLoLmt_rpm]
  EVCU2 SCP/2(VTQD_EVCU2MinTorqAvail_pct) -> [VTQD_EVCU2MinTorqAvail_pct]
  RC1 SCP/13(VTQD_RC1RefRetTrq_Nm) -> [VTQD_RC1RefRetTrq_Nm]
  [VTQD_EMRC1ActEMOutSftSpd_rpm] -> Bus Creator/15
  [VTQD_EMRC1EMTquModeDrvBrk_enum] -> Bus Creator/13
  [VTQD_EC1PercTorqIdleP5_pct] -> Bus Creator/26
  [VTQD_EMRC1ActEMpTrq_pct] -> Bus Creator/14
  [VTQD_EC1EMReqSpdCtrlLoLmt_rpm] -> Bus Creator/31
  [BInpConvert_outputs] -> ABS_System_Enable/1(BInpConvert_outputs)
  ADAS_DriverWheelTqDem/1(VTQD_ADASDriverDemWhTq_Nm) -> [VTQD_ADASDriverDemWhTq_Nm]
  RC1 SCP/4(VTQD_RC1RetSpdIdleP1_rpm) -> [VTQD_RC1RetSpdIdleP1_rpm]
  EC1 SCP/8(VTQD_EC1PercTorqIdleP4_pct) -> [VTQD_EC1PercTorqIdleP4_pct]
  [VTQD_EC1EMSupTSC1CtrlPG4_cnt] -> Bus Creator/42
  [VTQD_RC1PctTrqIdleP1_pct] -> Bus Creator/49
  [VTQD_EC1EMMaxMEngOvrSP7_rpm] -> Bus Creator/29
  [VTQD_RC1PctTrqPekTrqP5_pct] -> Bus Creator/55
  BMain_outputs/1 -> Terminator/1
  [VTQD_RC1RetSpdIdleP1_rpm] -> Bus Creator/48
  RC1 SCP/8(VTQD_RC1MaxRetSpdP3_rpm) -> [VTQD_RC1MaxRetSpdP3_rpm]
  MCUCMD SCP/3(VTQD_VCUMCUGearSta_enum) -> [VTQD_VCUMCUGearSta_enum]
  [BSCPIn_outputs] -> Buzzer Request/2(BSCPIn_outputs)
  EC1 SCP/4(VTQD_EC1PercTorqIdleP2_pct) -> [VTQD_EC1PercTorqIdleP2_pct]
  EC1 SCP/27(VTQD_EC1EMGainEndSpdGvn_gain) -> [VTQD_EC1EMGainEndSpdGvn_gain]
  [VTQD_EC1EMReqTrqCtrlUpLmt_pct] -> Bus Creator/34
  [VTQD_EC1EMSpdHdleP6_rpm] -> Bus Creator/43
  EMRC1 SCP/5(VTQD_EMRC1ActMaxAvaEMRecpTrq_pct) -> [VTQD_EMRC1ActMaxAvaEMRecpTrq_pct]
  [VTQD_RC1PctTrqP4_pct] -> Bus Creator/58
  [BInpConvert_outputs] -> Buzzer Request/1(BInpConvert_outputs)
  RC1 SCP/11(VTQD_RC1PctTrqP4_pct) -> [VTQD_RC1PctTrqP4_pct]
  [VTQD_VCUMCUGearSta_enum] -> Bus Creator/61
  EC1 SCP/20(VTQD_EC1EMDefTrqLmt_rpm) -> [VTQD_EC1EMDefTrqLmt_rpm]
  [VTQD_EEC3NFricPercTorq_pct] -> Bus Creator/10
  [VTQD_RC1RetSpdPekTrqP5_Nm] -> Bus Creator/59
  [VTQD_RC1PctTrqP3_pct] -> Bus Creator/53
  [VTQD_EC1EMRefTorq_Nm] -> Bus Creator/28
  [VTQD_ADASDriverDemWhTq_Nm] -> Bus Creator/62
  [VTQD_RC1RetCtrlMth_enum] -> Bus Creator/47
  [BInpConvert_outputs] -> TUpA Indication/1(BInpConvert_outputs)
  [VTQD_VCUMCUDemSpd_rpm] -> Bus Creator/60
  [VTQD_EMRC1ActMaxAvaEMRecpTrq_pct] -> Bus Creator/17
  [VTQD_RC1MaxRetSpdP2_rpm] -> Bus Creator/50
  EVCU1 SCP/6(VTQD_EVCU1EBrakeTorqLow_enum) -> [VTQD_EVCU1EBrakeTorqLow_enum]
  [VTQD_EC1PercTorqIdleP1_pct] -> Bus Creator/19
  [VTQD_EC1PercTorqIdleP3_pct] -> Bus Creator/23
  [VTQD_EC1EMSpdIdleP4_rpm] -> Bus Creator/24
  [VTQD_RC1RefRetTrq_Nm] -> Bus Creator/54
  [VTQD_TqReductEnable_flg] -> Bus Creator/64
  [VTQD_EC1EMDefTrqLmt_rpm] -> Bus Creator/37
  [VTQD_RC1RetType_enum] -> Bus Creator/45
  [VTQD_EC1EMMomOfInertia_kgpm2] -> Bus Creator/36
  [BSCPIn_outputs] -> ADAS_DriverWheelTqDem/2(BSCPIn_outputs)
  [VTQD_TUpAIND_enum] -> Bus Creator/65
  [VTQD_EC1EMSupTSC1CtrlPG1_cnt] -> Bus Creator/39
  Bus Creator/1 -> BOutpConvert_outputs/1  "BOutpConvert_outputs"
  [VTQD_EC1EMSupVarRTSC1MSG_cnt] -> Bus Creator/38
  [VTQD_EC1EMReqTrqCtrlLoLmt_pct] -> Bus Creator/32
  [VTQD_VCUBCMBuzzReq_flg] -> Bus Creator/66
  EC1 SCP/12(VTQD_EC1EMMaxMEngOvrSP7_rpm) -> [VTQD_EC1EMMaxMEngOvrSP7_rpm]
  EMRC1 SCP/4(VTQD_EMRC1ActEMpTrqHrls_pct) -> [VTQD_EMRC1ActEMpTrqHrls_pct]
  [VTQD_EVCU1EBrakeTorqLow_enum] -> Bus Creator/7
  RC1 SCP/1(VTQD_RC1RetType_enum) -> [VTQD_RC1RetType_enum]
  [VTQD_EVCU1EMotorSpd_rpm] -> Bus Creator/4
  RC1 SCP/10(VTQD_RC1RetSpdP4_rpm) -> [VTQD_RC1RetSpdP4_rpm]
  [VTQD_EVCU1EMotorPerformance_pct] -> Bus Creator/6
  MCUCMD SCP/1(VTQD_VCUMCUDemLoNegVal_rpm) -> [VTQD_VCUMCUDemLoNegVal_rpm]
  EC1 SCP/16(VTQD_EC1EMReqTrqCtrlLoLmt_pct) -> [VTQD_EC1EMReqTrqCtrlLoLmt_pct]
  RC1 SCP/12(VTQD_RC1RetSpdPekTrqP5_Nm) -> [VTQD_RC1RetSpdPekTrqP5_Nm]
  [VTQD_EEC3EMPressLoss_pct] -> Bus Creator/11
  [VTQD_EVCU1ActDrvMode_enum] -> Bus Creator/2
  [VTQD_VCUEBSHBSw_enum] -> Bus Creator/1
  Buzzer Request/1(VTQD_VCUBCMBuzzReq_flg) -> [VTQD_VCUBCMBuzzReq_flg]
  [VTQD_EVCU2MinTorqAvail_pct] -> Bus Creator/9
  [VTQD_EC1EMSpdIdleP1_rpm] -> Bus Creator/18
  [VTQD_EMRC1ActEMpTrqHrls_pct] -> Bus Creator/16
  EC1 SCP/6(VTQD_EC1PercTorqIdleP3_pct) -> [VTQD_EC1PercTorqIdleP3_pct]
  EC1 SCP/9(VTQD_EC1PercTorqIdleP5_pct) -> [VTQD_EC1PercTorqIdleP5_pct]
  EC1 SCP/11(VTQD_EC1EMRefTorq_Nm) -> [VTQD_EC1EMRefTorq_Nm]
  EC1 SCP/15(VTQD_EC1EMReqSpdCtrlUpLmt_rpm) -> [VTQD_EC1EMReqSpdCtrlUpLmt_rpm]
  ETC2 SCP/1(VTQD_ETC2ActDriveDirect_enum) -> [VTQD_ETC2ActDriveDirect_enum]
  EC1 SCP/17(VTQD_EC1EMReqTrqCtrlUpLmt_pct) -> [VTQD_EC1EMReqTrqCtrlUpLmt_pct]
  EC1 SCP/23(VTQD_EC1EMSupTSC1CtrlPG2_cnt) -> [VTQD_EC1EMSupTSC1CtrlPG2_cnt]
  EC1 SCP/24(VTQD_EC1EMSupTSC1CtrlPG3_cnt) -> [VTQD_EC1EMSupTSC1CtrlPG3_cnt]
  EC1 SCP/26(VTQD_EC1EMSpdHdleP6_rpm) -> [VTQD_EC1EMSpdHdleP6_rpm]
  EC1 SCP/18(VTQD_EC1EMExtRSCtrlUpLmt_rpm) -> [VTQD_EC1EMExtRSCtrlUpLmt_rpm]
  RC1 SCP/3(VTQD_RC1RetCtrlMth_enum) -> [VTQD_RC1RetCtrlMth_enum]
  EC1 SCP/5(VTQD_EC1EMSpdIdleP3_rpm) -> [VTQD_EC1EMSpdIdleP3_rpm]
  EC1 SCP/21(VTQD_EC1EMSupVarRTSC1MSG_cnt) -> [VTQD_EC1EMSupVarRTSC1MSG_cnt]
  RC1 SCP/5(VTQD_RC1PctTrqIdleP1_pct) -> [VTQD_RC1PctTrqIdleP1_pct]
  EC1 SCP/2(VTQD_EC1PercTorqIdleP1_pct) -> [VTQD_EC1PercTorqIdleP1_pct]
  [BInpConvert_outputs] -> ADAS_DriverWheelTqDem/1(BInpConvert_outputs)
  RC1 SCP/7(VTQD_RC1RetSpdP2_pct) -> [VTQD_RC1RetSpdP2_pct]
  MCUCMD SCP/2(VTQD_VCUMCUDemSpd_rpm) -> [VTQD_VCUMCUDemSpd_rpm]
  EVCU2 SCP/1(VTQD_EVCU2MaxTorqAvail_pct) -> [VTQD_EVCU2MaxTorqAvail_pct]
  RC1 SCP/6(VTQD_RC1MaxRetSpdP2_rpm) -> [VTQD_RC1MaxRetSpdP2_rpm]
  RC1 SCP/9(VTQD_RC1PctTrqP3_pct) -> [VTQD_RC1PctTrqP3_pct]
  ADAS_DriverWheelTqDem/2(VTQD_RealWhTq_Nm) -> [VTQD_RealWhTq_Nm]
  RC1 SCP/2(VTQD_RC1RetLocat_enum) -> [VTQD_RC1RetLocat_enum]
  EC1 SCP/19(VTQD_EC1EMMomOfInertia_kgpm2) -> [VTQD_EC1EMMomOfInertia_kgpm2]
  ABS_System_Enable/1(VTQD_TqReductEnable_flg) -> [VTQD_TqReductEnable_flg]
  TUpA Indication/1(VTQD_TUpAIND_enum) -> [VTQD_TUpAIND_enum]
  ETC1 SCP/1(VTQD_ETC1ShiftrPgs_enum) -> [VTQD_ETC1ShiftrPgs_enum]
  [VTQD_ETC1ShiftrPgs_enum] -> Bus Creator/67
  EVCU1 SCP/7(VTQD_EVCU1RecuperHighSta_enum) -> [VTQD_EVCU1RecuperHighSta_enum]
  [VTQD_EVCU1RecuperHighSta_enum] -> Bus Creator/68
  EMRC1 SCP/6(VTQD_EMRC1DrvDemEMRtapTrq_pct) -> [VTQD_EMRC1DrvDemEMRtapTrq_pct]
  EMRC1 SCP/7(VTQD_EMRC1RetSelNonEng_pct) -> [TQD_EMRC1RetSelNonEng_pct]
  EMRC1 SCP/8(VTQD_EMRC1SACtrlDev_cnt) -> [VTQD_EMRC1SACtrlDev_cnt]
  [VTQD_EMRC1DrvDemEMRtapTrq_pct] -> Bus Creator/69
  [TQD_EMRC1RetSelNonEng_pct] -> Bus Creator/70
  [VTQD_EMRC1SACtrlDev_cnt] -> Bus Creator/71
  [BInpConvert_outputs] -> MCUCMD SCP/2(BInpConvert_outputs)
  MCUCMD SCP/4(VTQD_VCUMCUHandBrk_flg) -> [VTQD_VCUMCUHandBrk_flg]
  MCUCMD SCP/5(VTQD_VCUMCUFootBrk_flg) -> [VTQD_VCUMCUFootBrk_flg]
  [VTQD_VCUMCUHandBrk_flg] -> Bus Creator/72
  [VTQD_VCUMCUFootBrk_flg] -> Bus Creator/73

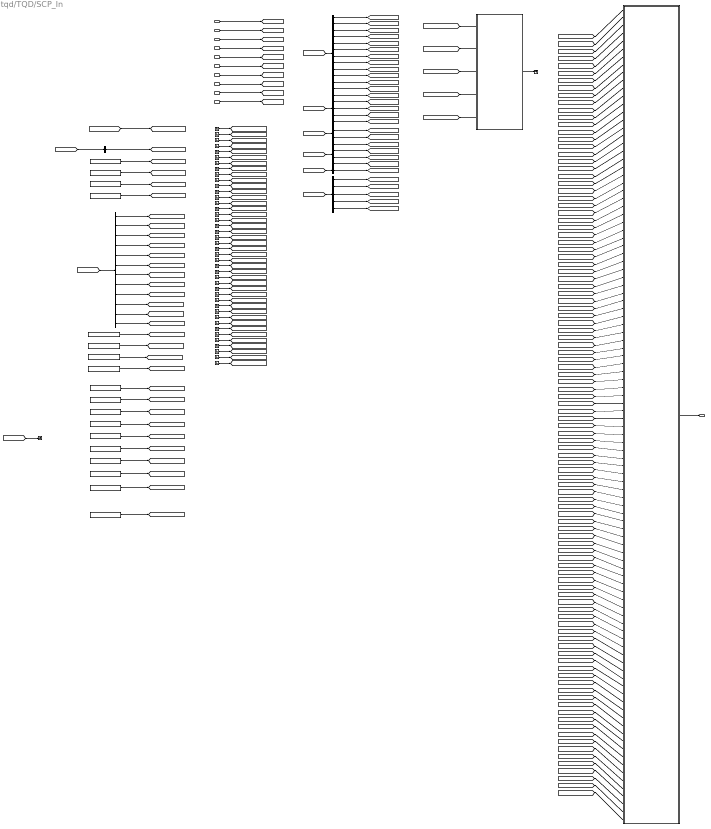
== system tqd/TQD/SCP_In ==
  note: From DID
  note: From CAN2
  note: %Reserved the vehicle Acceleration Limitaion form IVI/ECP.
      | @Acceleration Limiter
  note: From CAN3
  note: Fron CAN4
  note: %Singnal valid flg from INP libary.
      | @Acceleration Limiter, Speed Limiter, Invalid Condition
  note: From DDM
  note: From CAN1
  note: %Praking Brake Status form Zone digital pin.
      | @Combo Key, Parking Protection, Creep, Shift Modul, TUpA.
  note: %Driver seat belts stastus from Zone digitial pin.
      | @Parking Protection
  note: %Reserved for Masat front door status.
      | @SCP Door Status (Software Interoperability)
  note: %Reserved for Masat middle door status.
      | @SCP Door Status (Software Interoperability)
  note: %Reserved for Masat third door status.
      | @SCP Door Status (Software Interoperability)
  note: %Available charging current from BMS.
      | @Rolling Regen, Torque Capacity, EVCU1 SCP.
  note: %Singnal valid flg from INP libary.
      | @Creep, Accleration Limiter, Speed Limiter, Invalid Condition
  note: %Alarm coding form MCU.
      | @Creep
  note: %Systen fault level form @BMS.
      | @ECVU1 SCP
  note: %BMS pack  inner high voltage.
      | @Torque Capacity
  note: %BMS pack  output total current.
      | @Torque Capacity
  note: %Singnal valid flg from INP libary.
      | @Torque Capacity
  note: %Singnal valid flg from INP libary.
      | @Torque Capacity
  note: %MCU output torque upper limitation.
      | @Torque Capacity
  note: %MCU output torque lower limitation.
      | @Torque Capacity
  note: %Reserved the switch of Creep functuon form IVI/ECP.
      | @Creep
  note: %Reserved the vehicle Speed Limitaion form IVI/ECP.
      | @Speed Limiter
  note: %Reserved the switch of Speed Limiter functuon form IVI/ECP.
      | @Speed Limiter
  note: %Reserved the switch of Acceleration Limiter functuon form IVI/ECP.
      | @Speed Limiter
  note: %Reserved the switch of Speed Limiter functuon form IVI/ECP.
      | @Rolling Regen
  note: %Message valid flg.
      | @Rolling Regen
  note: %Message valid flg.
      | @Acceleration Limiter, Speed Limiter
  note: %Driving mode selection form IVI/ECP.
      | @Actual Driver Mode Determination
  note: %Door Safty function DID servise.
      | @Door Limit, Parking Protection.
  task_time_s : Inport
  BINP_CAN1_outputs : Inport  Port=2
  BINP_CAN2_outputs : Inport  Port=3
  BINP_CAN3_outputs : Inport  Port=4
  BINP_CAN4_outputs : Inport  Port=5
  BBCM_outputs : Inport  Port=6
  BDHP_outputs : Inport  Port=7
  BPMM_outputs : Inport  Port=8
  BPSA_outputs : Inport  Port=9
  BACC_outputs : Inport  Port=10
  Bus Selector : BusSelector  OutputSignals=VINP_EBSBrakeSw_enum,VINP_ASRHillHolderSw_enum,VINP_HillHolderMode_enum,VINP_TransReqGear_enum,VINP_BrakePedalPos_pct,VINP_EM1OvrCtrlMDriv_enum,VINP_EM1OvrCtrlMBrk_enum,VINP_EM1ReqTorqLimDriv_pct,VINP_EM1ReqTorqLimBrk_pct,VINP_CANMsgValidTC1_flg,VINP_FASpeed_kph,VINP_CANMsgValidEBC2_flg
  Bus Selector1 : BusSelector  OutputSignals=VINP_B2VAvaPlsChgCurr_A,VINP_MotorSpd_rpm,VINP_MotorTemp_C,VINP_MotorTrq_Nm,VINP_MCUFailGrade_enum,VINP_B2VSOC_pct,VINP_B2VAPlsDischgCurr_A,VINP_B2VFaultLv_enum,VINP_B2VPackInsideVol_V,VINP_B2VPackCurr_A,VINP_MCUTrqLimHi_Nm,VINP_MCUTrqLimLo_Nm
  Bus Selector2 : BusSelector  OutputSignals=VDHP_ActAPSPosn_pct,VDHP_LowIdleAccPedal_flg
  Bus Selector3 : BusSelector  OutputSignals=VBCM_FDCBCMFDoorSta_flg,VBCM_FDCBCMMDoorSta_flg,VBCM_FDCBCMFDOpenSVCmd_flg,VBCM_FDCBCMFDCloseSVCmd_flg,VBCM_FDCBCMRDoorSta_flg
  Bus Selector4 : BusSelector  OutputSignals=VPMM_DrivelineRelease_enum,VPMM_VCUMCUCtrlMd_enum,VPMM_SysPowerMode_enum,VPMM_PowerUpState_enum
  Bus Selector5 : BusSelector  OutputSignals=VPSA_Keystatus_enum
  Bus Selector6 : BusSelector  OutputSignals=VINP_ParkBrakeSW_enum
  Bus Selector7 : BusSelector  OutputSignals=VACC_ASC2KneeReqRSide_flg,VACC_ASC2KneeReqFA_flg,VACC_ASC2KneeReqRA_flg,VACC_ASC2NLvReqFA_enum,VACC_ASC2NLvReqRA_enum
  Constant12 : Constant  Value=KTQD_HVBPwrAvailDchrgValid_flg
  Constant13 : Constant  Value=KTQD_B2VAvaPlsChgCurrValid_flg
  Constant16 : Constant  Value=KTQD_ECPVCUCreepSW_flg
  Constant17 : Constant  Value=KTQD_ECPVCUSpdLim_kph
  Constant18 : Constant  Value=KTQD_ECPVCUSpdLimSw_flg
  Constant19 : Constant  Value=KTQD_ECPVCUAcclLim_mps
  Constant2 : Constant  Value=KTQD_SeatBeltSta_flg
  Constant20 : Constant  Value=KTQD_ECPVCUAcclLimSw_flg
  Constant21 : Constant  Value=KTQD_ECPVCURRegenSW_enum
  Constant22 : Constant  Value=KTQD_CANMsgValidECP3_flg
  Constant23 : Constant  Value=KTQD_CANMsgValidECP2_flg
  Constant24 : Constant  Value=KTQD_ECPVCUDRM_enum
  Constant3 : Constant  Value=KTQD_FRHalbrakeReq_enum
  Constant32 : Constant  Value=KTQD_DoorSaftySW_flg
  Constant4 : Constant  Value=KTQD_MDHalbrakeReq_enum
  Constant5 : Constant  Value=KTQD_TDHalbrakeReq_enum
  Constant7 : Constant  Value=KTQD_MotorSpdValid_flg
  Constant8 : Constant  Value=KTQD_MCUAlarmCode_cnt
  Ground{27..68} (42 alike) : Ground
  Input Signal : Subsystem
      settings: RTWSystemCode=Nonreusable function
  Invalid Condition : Subsystem
      settings: RTWSystemCode=Nonreusable function
  Terminator : Terminator
  Terminator1 : Terminator
  BSCPIn_outputs : Outport
  wires:
  Bus Selector1/2 -> [VINP_MotorSpd_rpm]  "<VINP_MotorSpd_rpm>"
  [VINP_MotorTrq_Nm] -> Input Signal/15(VINP_MotorTrq_Nm)
  [VINP_EBSBrakeSw_enum] -> Input Signal/2(VINP_EBSBrakeSw_enum)
  [VINP_FRHalbrakeReq_enum] -> Input Signal/34(VINP_FRHalbrakeReq_enum)
  Bus Selector2/1 -> [VDHP_ActAPSPosn_pct]  "<VDHP_ActAPSPosn_pct>"
  [VINP_ParkBrakeSW_flg] -> Input Signal/32(VINP_ParkBrakeSW_flg)
  Ground66/1 -> [VDMM_DTCDMSRCIncorrect_flg]
  [VINP_B2VSOC_pct] -> Input Signal/17(VINP_B2VSOC_pct)
  [VDMM_DTCEHPSInverNoFB_flg] -> Input Signal/88(VDMM_DTCEHPSInverNoFB_flg)
  [task_time_s] -> Input Signal/1(task_time_s)
  [VPMM_VCUMCUCtrlMd_enum] -> Input Signal/25(VPMM_VCUMCUCtrlMd_enum)
  [VINP_HillHolderMode_enum] -> Input Signal/4(VINP_HillHolderMode_enum)
  Ground67/1 -> [VDMM_MCURCIncorrect_flg]
  [VINP_EM1OvrCtrlMDriv_enum] -> Input Signal/7(VINP_EM1OvrCtrlMDriv_enum)
  [VINP_MotorSpdValid_flg] -> Input Signal/38(VINP_MotorSpdValid_flg)
  Bus Selector2/2 -> [VDHP_LowIdleAccPedal_flg]  "<VDHP_LowIdleAccPedal_flg>"
  Bus Selector/11 -> [VINP_FASpeed_kph]  "<VINP_FASpeed_kph>"
  Ground39/1 -> [VDMM_ActLostMCUSta1_flg]
  [VINP_EM1OvrCtrlMBrk_enum] -> Input Signal/8(VINP_EM1OvrCtrlMBrk_enum)
  [VDMM_DTCEBSCSIncorrect_flg] -> Input Signal/94(VDMM_DTCEBSCSIncorrect_flg)
  [VBCM_FDCBCMFDoorSta_flg] -> Input Signal/18(VBCM_FDCBCMFDoorSta_flg)
  [VINP_MCUFailGrade_enum] -> Input Signal/16(VINP_MCUFailGrade_enum)
  [VINP_ECPVCUSpdLimSw_flg] -> Input Signal/43(VINP_ECPVCUSpdLimSw_flg)
  Bus Selector4/3 -> [VPMM_SysPowerMode_enum]  "<VPMM_SysPowerMode_enum>"
  [VINP_TransReqGear_enum] -> Input Signal/5(VINP_TransReqGear_enum)
  [VDMM_DTCEBSRCIncorrect_flg] -> Invalid Condition/4(VDMM_DTCEBSRCIncorrect_flg)
  Ground33/1 -> [VDMM_DTCLostEBC2_flg]
  [VDMM_MCURCIncorrect_flg] -> Invalid Condition/1(VDMM_MCURCIncorrect_flg)
  Ground59/1 -> [VDMM_DTCEHPSRlyNoFB_flg]
  [VINP_BrakePedalPos_pct] -> Input Signal/6(VINP_BrakePedalPos_pct)
  [VINP_B2VAvaPlsChgCurr_A] -> Input Signal/37(VINP_B2VAvaPlsChgCurr_A)
  [VINP_ASRHillHolderSw_enum] -> Input Signal/3(VINP_ASRHillHolderSw_enum)
  [VINP_EM1ReqTorqLimBrk_pct] -> Input Signal/10(VINP_EM1ReqTorqLimBrk_pct)
  [VINP_FASpeed_kph] -> Input Signal/12(VINP_FASpeed_kph)
  [VINP_SeatBeltSta_flg] -> Input Signal/33(VINP_SeatBeltSta_flg)
  [VACC_ASC2NLvReqFA_enum] -> Input Signal/56(VACC_ASC2NLvReqFA_enum)
  Ground31/1 -> [VDMM_DTCLostEMCEM1_flg]
  [VINP_CANMsgValidECP3_flg] -> Input Signal/47(VINP_CANMsgValidECP3_flg)
  [VPMM_DrivelineRelease_enum] -> Input Signal/24(VPMM_DrivelineRelease_enum)
  [VINP_CANMsgValidTC1_flg] -> Input Signal/11(VINP_CANMsgValidTC1_flg)
  [VINP_EM1ReqTorqLimDriv_pct] -> Input Signal/9(VINP_EM1ReqTorqLimDriv_pct)
  Bus Selector/7 -> [VINP_EM1OvrCtrlMBrk_enum]  "<VINP_EM1OvrCtrlMBrk_enum>"
  [VINP_CANMsgValidECP2_flg] -> Input Signal/48(VINP_CANMsgValidECP2_flg)
  Ground47/1 -> [VDMM_DTCPDURCIncorrect_flg]
  [VINP_ECPVCUCreepSW_flg] -> Input Signal/41(VINP_ECPVCUCreepSW_flg)
  [VINP_MotorSpd_rpm] -> Input Signal/13(VINP_MotorSpd_rpm)
  Ground32/1 -> [VDMM_DTCLostEBC1_flg]
  [VPMM_PowerUpState_enum] -> Input Signal/27(VPMM_PowerUpState_enum)
  [VBCM_FDCBCMMDoorSta_flg] -> Input Signal/19(VBCM_FDCBCMMDoorSta_flg)
  [VBCM_FDCBCMRDoorSta_flg] -> Input Signal/54(VBCM_FDCBCMRDoorSta_flg)
  Ground48/1 -> [VDMM_DTCMCUCtrlMdNoFB_flg]
  [VDHP_ActAPSPosn_pct] -> Input Signal/22(VDHP_ActAPSPosn_pct)
  [VINP_MotorTemp_C] -> Input Signal/14(VINP_MotorTemp_C)
  [VINP_ECPVCURRegenSW_enum] -> Input Signal/46(VINP_ECPVCURRegenSW_enum)
  [VPMM_SysPowerMode_enum] -> Input Signal/26(VPMM_SysPowerMode_enum)
  [VDMM_ActLostEBC5_flg] -> Input Signal/68(VDMM_ActLostEBC5_flg)
  [VBCM_FDCBCMFDOpenSVCmd_flg] -> Input Signal/20(VBCM_FDCBCMFDOpenSVCmd_flg)
  [VINP_ECPVCUDRM_enum] -> Input Signal/49(VINP_ECPVCUDRM_enum)
  [VACC_ASC2KneeReqFA_flg] -> Input Signal/51(VACC_ASC2KneeReqFA_flg)
  [VDHP_LowIdleAccPedal_flg] -> Input Signal/23(VDHP_LowIdleAccPedal_flg)
  [VDMM_DTCMotorTrqNoFB_flg] -> Input Signal/90(VDMM_DTCMotorTrqNoFB_flg)
  [VINP_ECPVCUSpdLim_kph] -> Input Signal/42(VINP_ECPVCUSpdLim_kph)
  [VBCM_FDCBCMFDCloseSVCmd_flg] -> Input Signal/21(VBCM_FDCBCMFDCloseSVCmd_flg)
  [VINP_FASpeedValid_flg] -> Input Signal/31(VINP_FASpeedValid_flg)
  [VINP_MCUAlarmCode_cnt] -> Input Signal/39(VINP_MCUAlarmCode_cnt)
  [VACC_ASC2KneeReqRSide_flg] -> Input Signal/50(VACC_ASC2KneeReqRSide_flg)
  Ground35/1 -> [VDMM_ActLostEMCEM1_flg]
  Bus Selector3/4 -> [VBCM_FDCBCMFDCloseSVCmd_flg]  "<VBCM_FDCBCMFDCloseSVCmd_flg>"
  [VINP_ECPVCUAcclLim_mps] -> Input Signal/44(VINP_ECPVCUAcclLim_mps)
  [VPSA_Keystatus_enum] -> Input Signal/28(VPSA_Keystatus_enum)
  [VINP_MDHalbrakeReq_enum] -> Input Signal/35(VINP_MDHalbrakeReq_enum)
  [VINP_B2VFaultLv_enum] -> Input Signal/40(VINP_B2VFaultLv_enum)
  Ground61/1 -> [VDMM_DTCMotorSpdNoFB_flg]
  [VINP_TDHalbrakeReq_enum] -> Input Signal/36(VINP_TDHalbrakeReq_enum)
  Ground51/1 -> [VDMM_DTCBMSRlyNoFB_flg]
  [VINP_ECPVCUAcclLimSw_flg] -> Input Signal/45(VINP_ECPVCUAcclLimSw_flg)
  [VDMM_DTCLostEMCEM1_flg] -> Input Signal/61(VDMM_DTCLostEMCEM1_flg)
  [VACC_ASC2NLvReqRA_enum] -> Input Signal/53(VACC_ASC2NLvReqRA_enum)
  [VACC_ASC2KneeReqRA_flg] -> Input Signal/52(VACC_ASC2KneeReqRA_flg)
  [VDMM_DTCDMSRCIncorrect_flg] -> Invalid Condition/3(VDMM_DTCDMSRCIncorrect_flg)
  Bus Selector/10 -> [VINP_CANMsgValidTC1_flg]  "<VINP_CANMsgValidTC1_flg>"
  Ground41/1 -> [VDMM_ActLostMCUSta3_flg]
  [VDSC_DoorSaftySW_flg] -> Input Signal/55(VDSC_DoorSaftySW_flg)
  Bus Selector1/4 -> [VINP_MotorTrq_Nm]  "<VINP_MotorTrq_Nm>"
  [VDMM_ActLostMCUSta3_flg] -> Input Signal/71(VDMM_ActLostMCUSta3_flg)
  [VDMM_DTCLostB2VST1_flg] -> Input Signal/57(VDMM_DTCLostB2VST1_flg)
  [VDMM_DTCLostB2VST2_flg] -> Input Signal/58(VDMM_DTCLostB2VST2_flg)
  [VDMM_DTCLostB2VCurrentLimit_flg] -> Input Signal/59(VDMM_DTCLostB2VCurrentLimit_flg)
  [VDMM_DTCDoorStaError_flg] -> Input Signal/95(VDMM_DTCDoorStaError_flg)
  [VDMM_DTCLostTC1_flg] -> Input Signal/60(VDMM_DTCLostTC1_flg)
  [VDMM_ActLostEBC1_flg] -> Input Signal/66(VDMM_ActLostEBC1_flg)
  [VDMM_DTCLostEBC2_flg] -> Input Signal/63(VDMM_DTCLostEBC2_flg)
  [VDMM_ActLostEBC2_flg] -> Input Signal/67(VDMM_ActLostEBC2_flg)
  [VDMM_DTCLostEBC1_flg] -> Input Signal/62(VDMM_DTCLostEBC1_flg)
  [VDMM_DTCLostEBC5_flg] -> Input Signal/64(VDMM_DTCLostEBC5_flg)
  [VDMM_ActLostEMCEM1_flg] -> Input Signal/65(VDMM_ActLostEMCEM1_flg)
  [VDMM_ActLostMCUSta1_flg] -> Input Signal/69(VDMM_ActLostMCUSta1_flg)
  [VDMM_ActLostB2VST1_flg] -> Input Signal/72(VDMM_ActLostB2VST1_flg)
  [VDMM_ActLostB2VST2_flg] -> Input Signal/73(VDMM_ActLostB2VST2_flg)
  Ground50/1 -> [VDMM_DTCMCUHVRlyNoFB_flg]
  [VDMM_ActLostMCUSta2_flg] -> Input Signal/70(VDMM_ActLostMCUSta2_flg)
  [VDMM_ActLostB2VCurrentLimit_flg] -> Input Signal/74(VDMM_ActLostB2VCurrentLimit_flg)
  [VDMM_DTCPDURCIncorrect_flg] -> Input Signal/77(VDMM_DTCPDURCIncorrect_flg)
  [VDMM_DTCMCUCtrlMdNoFB_flg] -> Input Signal/78(VDMM_DTCMCUCtrlMdNoFB_flg)
  [VDMM_DTCMCUHVRlyNoFB_flg] -> Input Signal/80(VDMM_DTCMCUHVRlyNoFB_flg)
  [VDMM_CAN1BUSOFF_flg] -> Input Signal/75(VDMM_CAN1BUSOFF_flg)
  [VDMM_DTCMCUIGBNoFB_flg] -> Input Signal/79(VDMM_DTCMCUIGBNoFB_flg)
  [VDMM_DTCBCURCIncorrect_flg] -> Input Signal/76(VDMM_DTCBCURCIncorrect_flg)
  Ground60/1 -> [VDMM_DTCMotorTrqNoFB_flg]
  [VDMM_EBSRCIncorrect_flg] -> Input Signal/82(VDMM_EBSRCIncorrect_flg)
  [VDMM_DTCACHVRlyNoFB_flg] -> Input Signal/83(VDMM_DTCACHVRlyNoFB_flg)
  [VDMM_DTCBMSRlyNoFB_flg] -> Input Signal/81(VDMM_DTCBMSRlyNoFB_flg)
  [VDMM_DTCDCDCInverNoFB_flg] -> Input Signal/84(VDMM_DTCDCDCInverNoFB_flg)
  [VDMM_DTCDCDCRlyNoFB_flg] -> Input Signal/85(VDMM_DTCDCDCRlyNoFB_flg)
  [VDMM_DTCMotorSpdNoFB_flg] -> Input Signal/91(VDMM_DTCMotorSpdNoFB_flg)
  Bus Selector4/4 -> [VPMM_PowerUpState_enum]  "<VPMM_PowerUpState_enum>"
  [VDMM_DTCPBWireFailure_flg] -> Input Signal/92(VDMM_DTCPBWireFailure_flg)
  [VDMM_DTCEACRlyNoFB_flg] -> Input Signal/87(VDMM_DTCEACRlyNoFB_flg)
  [VDMM_DTCEHPSRlyNoFB_flg] -> Input Signal/89(VDMM_DTCEHPSRlyNoFB_flg)
  Ground49/1 -> [VDMM_DTCMCUIGBNoFB_flg]
  [VDMM_DTCEACInverNoFB_flg] -> Input Signal/86(VDMM_DTCEACInverNoFB_flg)
  Bus Selector5/1 -> [VPSA_Keystatus_enum]  "<VPSA_Keystatus_enum>"
  [VDMM_DTCDMSRCIncorrect_flg] -> Input Signal/96(VDMM_DTCDMSRCIncorrect_flg)
  [VDMM_MCURCIncorrect_flg] -> Input Signal/97(VDMM_MCURCIncorrect_flg)
  [VDMM_DTCBCMDoorStaLostCom_flg] -> Input Signal/93(VDMM_DTCBCMDoorStaLostCom_flg)
  [BBCM_outputs] -> Bus Selector3/1
  [VDMM_DTCEBSRCIncorrect_flg] -> Input Signal/98(VDMM_DTCEBSRCIncorrect_flg)
  Ground37/1 -> [VDMM_ActLostEBC2_flg]
  [BINP_CAN1_outputs] -> Bus Selector/1
  Bus Selector/8 -> [VINP_EM1ReqTorqLimDriv_pct]  "<VINP_EM1ReqTorqLimDriv_pct>"
  [BINP_CAN3_outputs] -> Bus Selector1/1
  Ground55/1 -> [VDMM_DTCDCDCRlyNoFB_flg]
  Bus Selector/4 -> [VINP_TransReqGear_enum]  "<VINP_TransReqGear_enum>"
  Bus Selector/5 -> [VINP_BrakePedalPos_pct]  "<VINP_BrakePedalPos_pct>"
  Bus Selector/2 -> [VINP_ASRHillHolderSw_enum]  "<VINP_ASRHillHolderSw_enum>"
  BDHP_outputs/1 -> [BDHP_outputs]
  Ground34/1 -> [VDMM_DTCLostEBC5_flg]
  Bus Selector/3 -> [VINP_HillHolderMode_enum]  "<VINP_HillHolderMode_enum>"
  Ground57/1 -> [VDMM_DTCEACRlyNoFB_flg]
  Bus Selector/6 -> [VINP_EM1OvrCtrlMDriv_enum]  "<VINP_EM1OvrCtrlMDriv_enum>"
  Bus Selector1/5 -> [VINP_MCUFailGrade_enum]  "<VINP_MCUFailGrade_enum>"
  Bus Selector1/3 -> [VINP_MotorTemp_C]  "<VINP_MotorTemp_C>"
  Bus Selector3/1 -> [VBCM_FDCBCMFDoorSta_flg]  "<VBCM_FDCBCMFDoorSta_flg>"
  Bus Selector/9 -> [VINP_EM1ReqTorqLimBrk_pct]  "<VINP_EM1ReqTorqLimBrk_pct>"
  Bus Selector3/2 -> [VBCM_FDCBCMMDoorSta_flg]  "<VBCM_FDCBCMMDoorSta_flg>"
  Bus Selector/1 -> [VINP_EBSBrakeSw_enum]  "<VINP_EBSBrakeSw_enum>"
  Bus Selector3/3 -> [VBCM_FDCBCMFDOpenSVCmd_flg]  "<VBCM_FDCBCMFDOpenSVCmd_flg>"
  Ground54/1 -> [VDMM_DTCDCDCInverNoFB_flg]
  Ground27/1 -> [VDMM_DTCLostB2VST1_flg]
  [BDHP_outputs] -> Bus Selector2/1
  Ground28/1 -> [VDMM_DTCLostB2VST2_flg]
  Ground29/1 -> [VDMM_DTCLostB2VCurrentLimit_flg]
  Ground30/1 -> [VDMM_DTCLostTC1_flg]
  Bus Selector4/2 -> [VPMM_VCUMCUCtrlMd_enum]  "<VPMM_VCUMCUCtrlMd_enum>"
  Ground58/1 -> [VDMM_DTCEHPSInverNoFB_flg]
  Bus Selector4/1 -> [VPMM_DrivelineRelease_enum]  "<VPMM_DrivelineRelease_enum>"
  [BPSA_outputs] -> Bus Selector5/1
  [BPMM_outputs] -> Bus Selector4/1
  Ground42/1 -> [VDMM_ActLostB2VST1_flg]
  Ground40/1 -> [VDMM_ActLostMCUSta2_flg]
  Ground38/1 -> [VDMM_ActLostEBC5_flg]
  Ground36/1 -> [VDMM_ActLostEBC1_flg]
  Invalid Condition/1(BDCQ_SCPInInValid_outputs) -> Terminator/1
  [VINP_FASpeedValid_flg] -> Invalid Condition/2(VINP_FASpeedValid_flg)
  Ground53/1 -> [VDMM_DTCACHVRlyNoFB_flg]
  Ground52/1 -> [VDMM_EBSRCIncorrect_flg]
  [VINP_MotorSpdValid_flg] -> Invalid Condition/5(VINP_MotorSpdValid_flg)
  Ground56/1 -> [VDMM_DTCEACInverNoFB_flg]
  Ground45/1 -> [VDMM_CAN1BUSOFF_flg]
  Ground46/1 -> [VDMM_DTCBCURCIncorrect_flg]
  Ground44/1 -> [VDMM_ActLostB2VCurrentLimit_flg]
  Ground43/1 -> [VDMM_ActLostB2VST2_flg]
  Ground68/1 -> [VDMM_DTCEBSRCIncorrect_flg]
  Ground62/1 -> [VDMM_DTCPBWireFailure_flg]
  Ground63/1 -> [VDMM_DTCBCMDoorStaLostCom_flg]
  Ground65/1 -> [VDMM_DTCDoorStaError_flg]
  Ground64/1 -> [VDMM_DTCEBSCSIncorrect_flg]
  Bus Selector1/6 -> [VINP_B2VSOC_pct]  "<VINP_B2VSOC_pct>"
  Input Signal/1(BSCP_In_outputs) -> BSCPIn_outputs/1  "BSCPIn_outputs"
  BPMM_outputs/1 -> [BPMM_outputs]
  BINP_CAN1_outputs/1 -> [BINP_CAN1_outputs]
  BINP_CAN3_outputs/1 -> [BINP_CAN3_outputs]
  BBCM_outputs/1 -> [BBCM_outputs]
  BINP_CAN2_outputs/1 -> [BINP_CAN2_outputs]
  BINP_CAN4_outputs/1 -> [BINP_CAN4_outputs]
  task_time_s/1 -> [task_time_s]
  BPSA_outputs/1 -> [BPSA_outputs]
  Bus Selector/12 -> [VINP_CANMsgValidEBC2_flg]  "<VINP_CANMsgValidEBC2_flg>"
  [VINP_CANMsgValidEBC2_flg] -> Input Signal/29(VINP_CANMsgValidEBC2_flg)
  Bus Selector1/7 -> [VINP_B2VAPlsDischgCurr_A]  "<VINP_B2VAPlsDischgCurr_A>"
  [VINP_B2VAPlsDischgCurr_A] -> Input Signal/30(VINP_B2VAPlsDischgCurr_A)
  [VINP_B2VAvaPlsChgCurrValid_flg] -> Input Signal/102(VINP_B2VAvaPlsChgCurrValid_flg)
  [VINP_HVBPwrAvailDchrgValid_flg] -> Input Signal/101(VINP_HVBPwrAvailDchrgValid_flg)
  [VINP_B2VPackCurr_A] -> Input Signal/100(VINP_B2VPackCurr_A)
  [VINP_B2VPackInsideVol_V] -> Input Signal/99(VINP_B2VPackInsideVol_V)
  [VINP_MCUTrqLimHi_Nm] -> Input Signal/103(VINP_MCUTrqLimHi_Nm)
  [VINP_MCUTrqLimLo_Nm] -> Input Signal/104(VINP_MCUTrqLimLo_Nm)
  [BINP_CAN4_outputs] -> Bus Selector6/1
  [VINP_CANMsgValidEBC2_flg] -> [VINP_FASpeedValid_flg]
  Bus Selector6/1 -> [VINP_ParkBrakeSW_flg]  "<VINP_ParkBrakeSW_enum>"
  Constant2/1 -> [VINP_SeatBeltSta_flg]
  Constant3/1 -> [VINP_FRHalbrakeReq_enum]
  Constant4/1 -> [VINP_MDHalbrakeReq_enum]
  Constant5/1 -> [VINP_TDHalbrakeReq_enum]
  Bus Selector1/1 -> [VINP_B2VAvaPlsChgCurr_A]  "<VINP_B2VAvaPlsChgCurr_A>"
  Constant7/1 -> [VINP_MotorSpdValid_flg]
  Constant8/1 -> [VINP_MCUAlarmCode_cnt]
  Bus Selector1/8 -> [VINP_B2VFaultLv_enum]  "<VINP_B2VFaultLv_enum>"
  Bus Selector1/9 -> [VINP_B2VPackInsideVol_V]  "<VINP_B2VPackInsideVol_V>"
  Bus Selector1/10 -> [VINP_B2VPackCurr_A]  "<VINP_B2VPackCurr_A>"
  Constant12/1 -> [VINP_HVBPwrAvailDchrgValid_flg]
  Constant13/1 -> [VINP_B2VAvaPlsChgCurrValid_flg]
  Bus Selector1/11 -> [VINP_MCUTrqLimHi_Nm]  "<VINP_MCUTrqLimHi_Nm>"
  Bus Selector1/12 -> [VINP_MCUTrqLimLo_Nm]  "<VINP_MCUTrqLimLo_Nm>"
  Constant16/1 -> [VINP_ECPVCUCreepSW_flg]
  Constant17/1 -> [VINP_ECPVCUSpdLim_kph]
  Constant18/1 -> [VINP_ECPVCUSpdLimSw_flg]
  Constant19/1 -> [VINP_ECPVCUAcclLim_mps]
  Constant20/1 -> [VINP_ECPVCUAcclLimSw_flg]
  Constant21/1 -> [VINP_ECPVCURRegenSW_enum]
  Constant22/1 -> [VINP_CANMsgValidECP3_flg]
  Constant23/1 -> [VINP_CANMsgValidECP2_flg]
  Constant24/1 -> [VINP_ECPVCUDRM_enum]
  Constant32/1 -> [VDSC_DoorSaftySW_flg]
  [BINP_CAN2_outputs] -> Terminator1/1
  Bus Selector3/5 -> [VBCM_FDCBCMRDoorSta_flg]  "<VBCM_FDCBCMRDoorSta_flg>"
  BACC_outputs/1 -> [BACC_outputs]
  [BACC_outputs] -> Bus Selector7/1
  Bus Selector7/1 -> [VACC_ASC2KneeReqRSide_flg]  "<VACC_ASC2KneeReqRSide_flg>"
  Bus Selector7/2 -> [VACC_ASC2KneeReqFA_flg]  "<VACC_ASC2KneeReqFA_flg>"
  Bus Selector7/3 -> [VACC_ASC2KneeReqRA_flg]  "<VACC_ASC2KneeReqRA_flg>"
  Bus Selector7/4 -> [VACC_ASC2NLvReqFA_enum]  "<VACC_ASC2NLvReqFA_enum>"
  Bus Selector7/5 -> [VACC_ASC2NLvReqRA_enum]  "<VACC_ASC2NLvReqRA_enum>"
